simulink model "flextemplate"  (Simulink 7.8)
settings: Solver=ode45  StartTime=0.0  StopTime=5  RelTol=1e-3
values from neighbouring files (symbols this model uses):
  h = 0.1    [linid.m]    (also in nonlinid.m = 0.05)
settings Model: Creator=rbabuska  LastModifiedBy=rbabuska
settings OptimizationCC: InitFltsAndDblsToZero=on
settings DebuggingCC: SaveWithParameterizedLinksMsg=none  SignalResolutionControl=TryResolveAllWithWarning  MultiTaskCondExecSysMsg=none  FcnCallInpInsideContextMsg=Use local settings  StrictBusMsg=Warning
settings RTWCC: IncludeERTFirstTime=on
settings GRTTargetCC: TargetFcnLib=ansi_tfl_tmw.mat

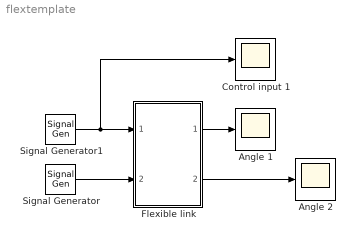
== system flextemplate ==
  Angle 1 : Scope
      settings: TimeRange=5  YMin=-25  SaveName=y1  DataFormat=Array  SampleInput=on  SampleTime=h
  Angle 2 : Scope
      settings: TimeRange=5  YMin=-25  SaveName=y  DataFormat=Array  SampleInput=on  SampleTime=h
  Control input 1 : Scope
      settings: TimeRange=5  YMin=-0.5  YMax=0.5  SaveName=u1  DataFormat=Array  SampleInput=on  SampleTime=h
  Flexible link : Subsystem  mask{Ts=h}
      mask prompts: Ts "Sampling period"
      mask Display: disp('Flexible link')
  Signal Generator : SignalGenerator  Amplitude=0  Frequency=2
  Signal Generator1 : SignalGenerator  WaveForm=square  Amplitude=.5
  wires:
  Signal Generator1/1 -> Flexible link/1(Input 1), Control input 1/1
  Flexible link/1(Angle 1) -> Angle 1/1
  Flexible link/2(Angle 2) -> Angle 2/1
  Signal Generator/1 -> Flexible link/2(Input 2)

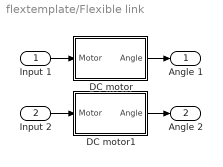
== system flextemplate/Flexible link ==
  Input 1 : Inport
  Input 2 : Inport  Port=2
  DC motor : Subsystem  mask{h=Ts, setupnr=1}
      mask prompts: h "Sample time [s]:"; setupnr "Setup number (for instance 1 or 2, etc.)"
      mask Display: disp('DC Motor')
  DC motor1 : Subsystem  mask{h=Ts, setupnr=2}
      mask prompts: h "Sample time [s]:"; setupnr "Setup number (for instance 1 or 2, etc.)"
      mask Display: disp('DC Motor')
  Angle 1 : Outport
  Angle 2 : Outport  Port=2
  wires:
  Input 1/1 -> DC motor/1(Motor)
  DC motor/1(Angle) -> Angle 1/1
  Input 2/1 -> DC motor1/1(Motor)
  DC motor1/1(Angle) -> Angle 2/1

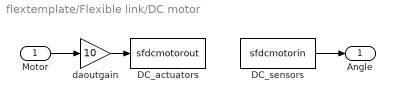
== system flextemplate/Flexible link/DC motor ==
  Motor : Inport
  DC_actuators : S-Function  FunctionName=sfdcmotorout  Parameters=Ts, H  EnableBusSupport=off  mask(Serial Out){Ts=h, setupnr=setupnr}
      mask prompts: Ts "Sample time:"; setupnr "Setup number:"
      mask help: Serial line output block
      mask init:
      | H=fugiboard('Open', ['mops' num2str(setupnr)]);
      mask Help: Serial Out block is designed as a serial communication output block for real time data acquisition, signal processing and control applications.
      mask Display: disp('DC Motor');
  DC_sensors : S-Function  FunctionName=sfdcmotorin  Parameters=Ts, H  EnableBusSupport=off  mask(Serial Out){Ts=h, setupnr=setupnr}
      mask prompts: Ts "Sample time:"; setupnr "Setup number"
      mask help: Serial line output block
      mask init:
      | H=fugiboard('Open', ['mops' num2str(setupnr)]);
      mask Help: Serial Out block is designed as a serial communication output block for real time data acquisition, signal processing and control applications.
      mask Display: disp('DC Motor');
  daoutgain : Gain  Gain=10  SaturateOnIntegerOverflow=on  OutDataTypeStr=Inherit: Same as input  ParamDataTypeStr=Inherit: Same as input
  Angle : Outport
  wires:
  Motor/1 -> daoutgain/1
  DC_sensors/1 -> Angle/1
  daoutgain/1 -> DC_actuators/1

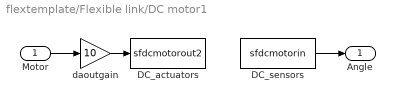
== system flextemplate/Flexible link/DC motor1 ==
  Motor : Inport
  DC_actuators : S-Function  FunctionName=sfdcmotorout2  Parameters=Ts, H  EnableBusSupport=off  mask(Serial Out){Ts=h, setupnr=setupnr}
      mask prompts: Ts "Sample time:"; setupnr "Setup number:"
      mask help: Serial line output block
      mask init:
      | H=fugiboard('Open', ['mops' num2str(setupnr)]);
      mask Help: Serial Out block is designed as a serial communication output block for real time data acquisition, signal processing and control applications.
      mask Display: disp('DC Motor');
  DC_sensors : S-Function  FunctionName=sfdcmotorin  Parameters=Ts, H  EnableBusSupport=off  mask(Serial Out){Ts=h, setupnr=setupnr}
      mask prompts: Ts "Sample time:"; setupnr "Setup number"
      mask help: Serial line output block
      mask init:
      | H=fugiboard('Open', ['mops' num2str(setupnr)]);
      mask Help: Serial Out block is designed as a serial communication output block for real time data acquisition, signal processing and control applications.
      mask Display: disp('DC Motor');
  daoutgain : Gain  Gain=10  SaturateOnIntegerOverflow=on  OutDataTypeStr=Inherit: Same as input  ParamDataTypeStr=Inherit: Same as input
  Angle : Outport
  wires:
  daoutgain/1 -> DC_actuators/1
  DC_sensors/1 -> Angle/1
  Motor/1 -> daoutgain/1
